simulink model "denemeForGlobal"  (R2015a)
settings: Solver=ode45  StartTime=0.0  StopTime=10.0  RelTol=1e-3
settings Model: Creator=Administrator  LastModifiedBy=Administrator

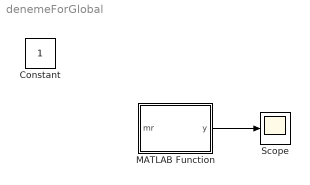
== system denemeForGlobal ==
  Constant : Constant
  MATLAB Function : MATLAB Function  TreatAsAtomicUnit=on
  Scope : Scope
  wires:
  MATLAB Function/1(y) -> Scope/1

== matlab function denemeForGlobal/MATLAB Function ==
  data: y output; mr input
function y = fcn(mr)
y=mr;
